simulink model "Subsystem"  (R2020b)
settings: Solver=FixedStepAuto  StartTime=0.0  StopTime=10.0  FixedStep=1  RelTol=1e-3
settings Model: Creator=Pulkit Khandelwal  LastModifiedBy=Pulkit Khandelwal
settings DataIOCC: SaveOutput=off  SaveTime=off

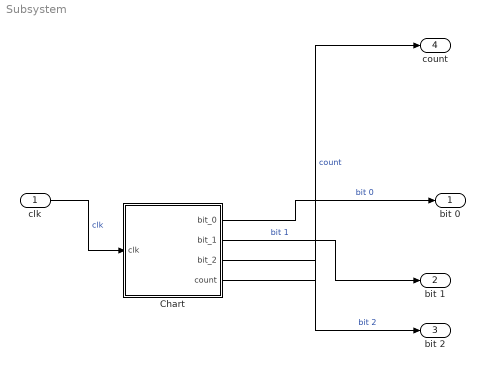
== system Subsystem ==
  clk : Inport  OutDataTypeStr=double  PortDimensions=1  SampleTime=[1,0]
  Chart : Stateflow chart  TreatAsAtomicUnit=on
  bit 0 : Outport  OutDataTypeStr=double  PortDimensions=1  SampleTime=[1,0]
  bit 1 : Outport  Port=2  OutDataTypeStr=double  PortDimensions=1  SampleTime=[1,0]
  bit 2 : Outport  Port=3  OutDataTypeStr=double  PortDimensions=1  SampleTime=[1,0]
  count : Outport  Port=4  OutDataTypeStr=double  PortDimensions=1  SampleTime=[1,0]
  wires:
  clk/1 -> Chart/1(clk)  "clk"
  Chart/2(bit_1) -> bit 1/1  "bit 1"
  Chart/1(bit_0) -> bit 0/1  "bit 0"
  Chart/3(bit_2) -> bit 2/1  "bit 2"
  Chart/4(count) -> count/1  "count"

== stateflow chart Subsystem/Chart ==
  state STATE0
    entry:
    bit_0 = 0;
    bit_1 = 0;
    bit_2 = 0;
    exit:
    count = 0;
  state STATE1
    entry:
    bit_0 =1;
    bit_1 = 0;
    bit_2 = 0;
    exit:
    count = 1;
  state STATE5
    entry:
    bit_0=0;
    bit_1=0;
    bit_2=1;
    exit:
    count = 4;
  state STATE2
    entry:
    bit_0 = 0;
    bit_1 = 1;
    bit_2 =0;
    exit:
    count=2;
  state STATE3
    entry:
    bit_0 =1;
    bit_1 =1;
    bit_2 = 0;
    exit:
    count=3;
  (default) -> STATE0
  STATE5 -> STATE0 : [clk==1]
  STATE0 -> STATE1 : [clk==1]
  STATE1 -> STATE2 : [clk==1]
  STATE3 -> STATE5 : [clk==1]
  STATE2 -> STATE3 : [clk==1]
  data: clk input; bit_0 output; bit_1 output; bit_2 output; count output
